simulink model "HW4_3"  (R2023a)
settings: Solver=VariableStepAuto  StartTime=0.0  StopTime=50  RelTol=1e-3
settings Model: Creator=BRL  LastModifiedBy=BRL

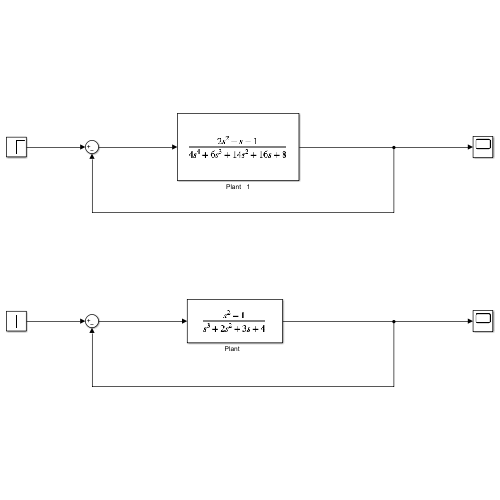
[thumbnail: Simulink's stored preview of the top-level diagram]
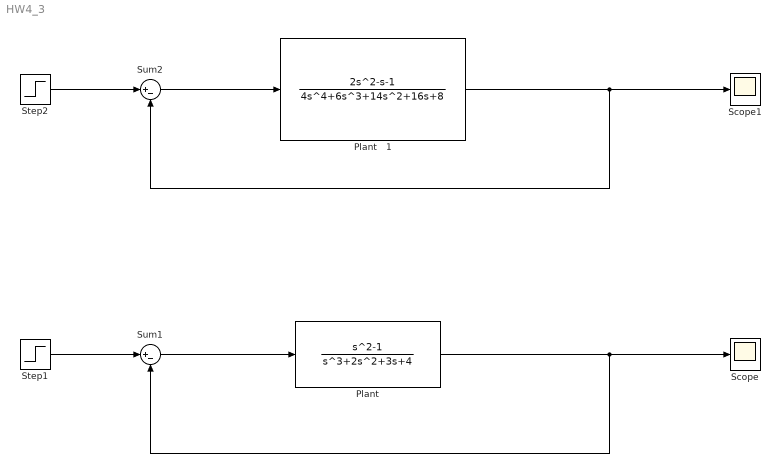
== system HW4_3 ==
  "Plant   " : TransferFcn  Numerator=[0 1 0 -1]  Denominator=[1 2 3 4]
  Plant   1 : TransferFcn  Numerator=[0 0 2 -1 -1]  Denominator=[4 6 14 16 8]
  Scope : Scope
  Scope1 : Scope
  Step1 : Step  SampleTime=0
  Step2 : Step  SampleTime=0
  Sum1 : Sum  Inputs=|+-
  Sum2 : Sum  Inputs=|+-
  wires:
  "Plant   "/1 -> Scope/1, Sum1/2
  Step1/1 -> Sum1/1
  Sum1/1 -> "Plant   "/1
  Plant   1/1 -> Scope1/1, Sum2/2
  Sum2/1 -> Plant   1/1
  Step2/1 -> Sum2/1
